simulink model "car"  (R2018a)
settings: Solver=VariableStepAuto  StartTime=0.0  StopTime=10  RelTol=1e-3
model workspace (MAT data in the model file):
  PAC1996coefficients = 0
undefined symbols (not defined in the file or in its folder): sigbuilder_block
libraries: simulink_extras x5, CarLib x2, simulink x1
settings Model: Creator=Seb  LastModifiedBy=PolimarcheRacingTeam

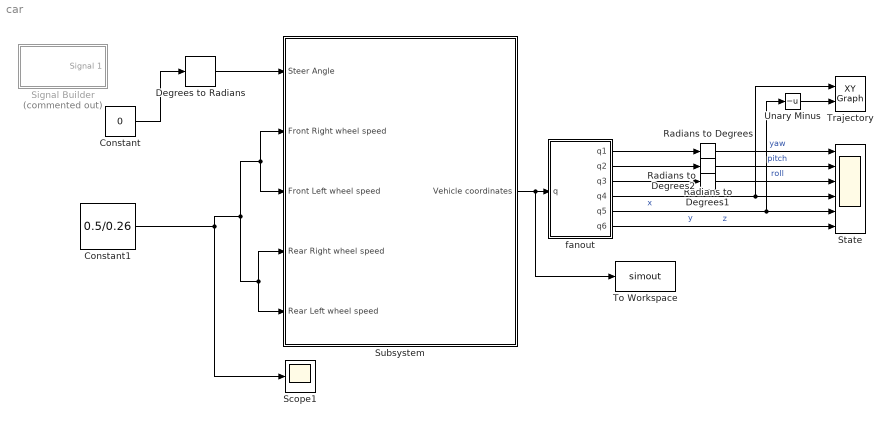
== system car ==
  Constant : Constant  Value=0
  Constant1 : Constant  Value=0.5/0.26
  Degrees to Radians : simulink_extras/Transformations/Degrees to Radians
  Radians to Degrees : simulink_extras/Transformations/Radians to Degrees
  Radians to Degrees1 : simulink_extras/Transformations/Radians to Degrees
  Radians to Degrees2 : simulink_extras/Transformations/Radians to Degrees
  Scope1 : Scope
  Signal Builder : Subsystem  Tag=STV Subsys  Commented=on  LoadFcn=sigbuilder_block('load');  StartFcn=sigbuilder_block('start');  StopFcn=sigbuilder_block('stop');  ClipboardFcn=sigbuilder_block('clipboard');  mask(Sigbuilder block){tuvar=[0:10]}
      mask help: Simulink:masks:SigbuilderBlock_MD
      mask init:
      | if ~strcmp(get_param(bdroot(gcbh),'SimulationStatus'),'stopped') tuvar = sigbuilder_block('maskInit'); end
      settings: CopyFcn=sigbuilder_block('copy');  DeleteFcn=sigbuilder_block('delete');  ModelCloseFcn=sigbuilder_block('modelClose');  PreSaveFcn=sigbuilder_block('preSave');  PauseFcn=sigbuilder_block('pause');  ContinueFcn=sigbuilder_block('continue');  NameChangeFcn=sigbuilder_block('namechange');  OpenFcn=sigbuilder_block('open',[240 166.5 550.5 399.75 ]);  CloseFcn=sigbuilder_block('close');
      mask Display: plot(0, 0, 100, 100,[2, 2, 32, 32, 2], [68, 8, 8, 68, 68],[32, 2], [38, 38], [32, 19, 2],[53, 60, 44], [32, 17, 17, 2],[16, 16, 31, 31]);txt = getActiveGroup(gcbh);text(2, 100, txt,'verticalAlignment', 'top');
  State : Scope  NumInputPorts=6
  Subsystem : Subsystem
  To Workspace : ToWorkspace  VariableName=simout  SaveFormat=Timeseries  SampleTime=-1
  Trajectory : simulink/Sinks/XY Graph  xmin=-1  xmax=20  ymin=-10  ymax=10  st=-1
  Unary Minus : UnaryMinus
  fanout : MATLAB Function  TreatAsAtomicUnit=on
  wires:
  fanout/2(q2) -> Radians to Degrees1/1
  fanout/3(q3) -> Radians to Degrees2/1
  fanout/4(q4) -> State/4, Trajectory/1  "x"
  fanout/6(q6) -> State/6  "z"
  fanout/1(q1) -> Radians to Degrees/1
  fanout/5(q5) -> State/5, Unary Minus/1  "y"
  Subsystem/1(Vehicle coordinates) -> To Workspace/1, fanout/1(q)
  Constant1/1 -> Subsystem/3(Front Left wheel speed), Subsystem/2(Front Right wheel speed), Subsystem/5(Rear Left wheel speed), Subsystem/4(Rear Right wheel speed), Scope1/1
  Unary Minus/1 -> Trajectory/2
  Radians to Degrees1/1 -> State/2  "pitch"
  Radians to Degrees2/1 -> State/3  "roll"
  Radians to Degrees/1 -> State/1  "yaw"
  Constant/1 -> Degrees to Radians/1
  Degrees to Radians/1 -> Subsystem/1(Steer Angle)

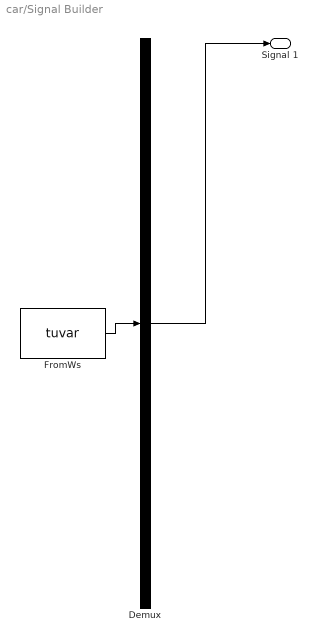
== system car/Signal Builder ==
  Demux : Demux  Tag=STV Demux  Outputs=1
  FromWs : FromWorkspace  Tag=STV FromWs  VariableName=tuvar  SampleTime=0
      SigBuilderData=|
      | common.afterFinalStr = 'Extrapolate'
      | common.sampleTime = 0
      | dataSet.timeRange = [0 10]
      | dataSet.name = 'Group 1'
      | sbobj.Groups.Name = 'Group 1'
      | sbobj.Groups.Signals.Name = 'Signal 1'
      | sbobj.Groups.Signals.XData = [0 1 4 4 6 6 8 10]
      | sbobj.Groups.Signals.YData = [0 0 8.2 8.18 8.18 8.05 0 0]
  Signal 1 : Outport  Tag=STV Outport
  wires:
  Demux/1 -> Signal 1/1
  FromWs/1 -> Demux/1

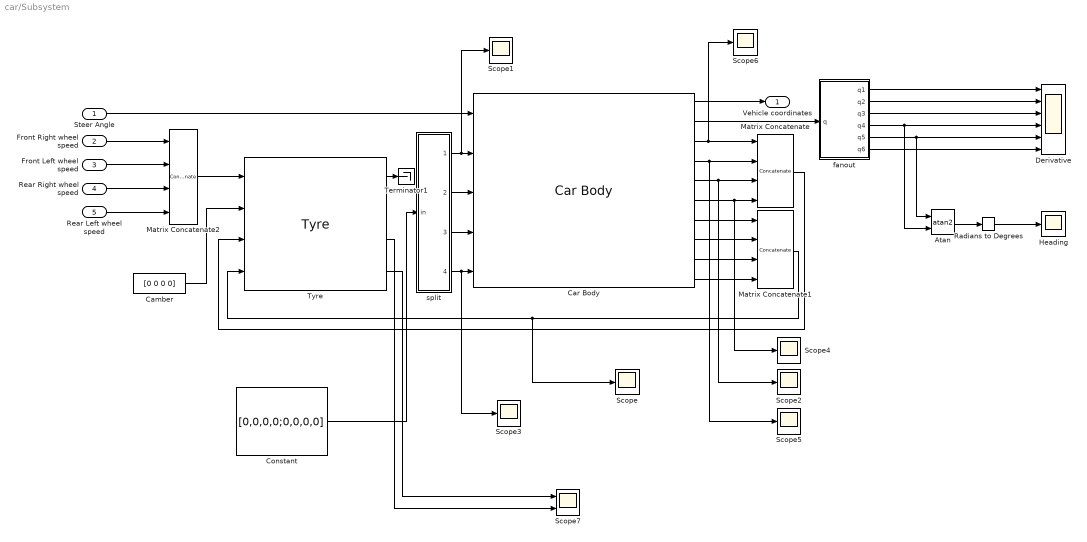
== system car/Subsystem ==
  Steer Angle : Inport  PortDimensions=1
  Front Right wheel speed : Inport  Port=2
  Front Left wheel speed : Inport  Port=3
  Rear Right wheel speed : Inport  Port=4
  Rear Left wheel speed : Inport  Port=5
  Atan : Trigonometry  Operator=atan2
  Camber : Constant  Value=[0 0 0 0]  VectorParams1D=off
  Car Body : CarLib/Car Body  x0="[0;-0.00445;0;  0;0;-0.287;  0;0;0;  1;1;0]"  paramsfile='myparams.mat'
  Constant : Constant  Value=[0,0,0,0;0,0,0,0]
  Derivative : Scope  NumInputPorts=6
  Heading : Scope
  Matrix Concatenate : Concatenate  NumInputs=4  Mode=Multidimensional array  ConcatenateDimension=2
  Matrix Concatenate1 : Concatenate  NumInputs=4  Mode=Multidimensional array  ConcatenateDimension=2
  Matrix Concatenate2 : Concatenate  NumInputs=4  Mode=Multidimensional array  ConcatenateDimension=2
  Radians to Degrees : simulink_extras/Transformations/Radians to Degrees
  Scope{,1..6} (7 alike) : Scope
  Scope7 : Scope  NumInputPorts=2
  Terminator1 : Terminator
  "Tyre " : CarLib/Tyre  tirfilename='Hoosier_43129_7inch_Round3.tir'
  fanout : MATLAB Function  TreatAsAtomicUnit=on
  split : MATLAB Function  TreatAsAtomicUnit=on
  Vehicle coordinates : Outport
  wires:
  Steer Angle/1 -> Car Body/1
  Car Body/10 -> Matrix Concatenate1/4
  Rear Left wheel speed/1 -> Matrix Concatenate2/4
  split/4(col4) -> Scope3/1, Car Body/5
  Car Body/9 -> Matrix Concatenate1/3
  Matrix Concatenate2/1 -> "Tyre "/1
  split/2(col2) -> Car Body/3
  Matrix Concatenate1/1 -> Scope/1, "Tyre "/4
  split/1(col1) -> Scope1/1, Car Body/2
  split/3(col3) -> Car Body/4
  Front Left wheel speed/1 -> Matrix Concatenate2/2
  Car Body/8 -> Matrix Concatenate1/2
  Car Body/7 -> Matrix Concatenate1/1
  Front Right wheel speed/1 -> Matrix Concatenate2/1
  Car Body/5 -> Scope2/1, Matrix Concatenate/3
  Rear Right wheel speed/1 -> Matrix Concatenate2/3
  Car Body/3 -> Scope6/1, Matrix Concatenate/1
  Car Body/4 -> Scope5/1, Matrix Concatenate/2
  Car Body/6 -> Scope4/1, Matrix Concatenate/4
  Car Body/1 -> Vehicle coordinates/1
  Camber/1 -> "Tyre "/2
  Matrix Concatenate/1 -> "Tyre "/3
  Car Body/2 -> fanout/1(q)
  Atan/1 -> Radians to Degrees/1
  fanout/5(q5) -> Derivative/5, Atan/1
  fanout/4(q4) -> Derivative/4, Atan/2
  fanout/1(q1) -> Derivative/1
  fanout/2(q2) -> Derivative/2
  fanout/3(q3) -> Derivative/3
  fanout/6(q6) -> Derivative/6
  "Tyre "/1 -> Terminator1/1
  Radians to Degrees/1 -> Heading/1
  "Tyre "/4 -> Scope7/1
  "Tyre "/3 -> Scope7/2
  Constant/1 -> split/1(in)

== matlab function car/fanout ==
  data: q1 output; q2 output; q3 output; q4 output; q input; q5 output; q6 output
function [q1,q2,q3,q4,q5,q6] = fanout(q)
    q1 = q(1);
    q2 = q(2);
    q3 = q(3);
    q4 = q(4);
    q5 = q(5);
    q6 = q(6);
end

== matlab function car/Subsystem/fanout ==
  data: q1 output; q2 output; q3 output; q4 output; q input; q5 output; q6 output
function [q1,q2,q3, q4,q5,q6] = fanout(q)
    q1 = q(1);
    q2 = q(2);
    q3 = q(3);
    q4 = q(4);
    q5 = q(5);
    q6 = q(6);
end

== matlab function car/Subsystem/split ==
  data: in input; col1 output; col2 output; col3 output; col4 output
function [col1,col2,col3,col4] = split(in)
    col1 = in(:,1);
    col2 = in(:,2);
    col3 = in(:,3);
    col4 = in(:,4);
end
